simulink model "step_model"  (R2015b)
settings: Solver=VariableStepAuto  StartTime=0.0  StopTime=10.0  RelTol=1e-3
values from neighbouring files (symbols this model uses):
  A = [zeros(2) eye(2); -inv(M)*kappa -inv(M)*beta]    [Lab3_Solution.m]    (also in lab4.m = [0 0 1 0; 0 0 0 1; 0 (mp^2 * l^2 *g)/mu (-c*Jt)/mu (-Y*Jt*l*; lab4_pid_controller.m; lab4_state_feedback_no_estimator.m; lab4_state_feedback_with_estimator.m)
  B = [0; 0; inv(M)*S]    [Lab3_Solution.m]    (also in lab4.m = [0; 0; Jt/mu; (l*mp)/mu]; lab4_pid_controller.m; lab4_state_feedback_no_estimator.m; lab4_state_feedback_with_estimator.m)
  C = [1 0 0 0; 0 1 0 0]    [Lab3_Solution.m]    (also in PendulumTutorial.m = zpk(z,p,k); lab4.m; lab4_pid_controller.m; lab4_state_feedback_no_estimator.m = eye(4))
  D = [0; 0]    [Lab3_Solution.m]    (also in lab4.m; lab4_pid_controller.m; lab4_state_feedback_no_estimator.m = [0; 0; 0; 0]; lab4_state_feedback_with_estimator.m)
settings Model: Creator=lukasgemar  LastModifiedBy=lukasgemar

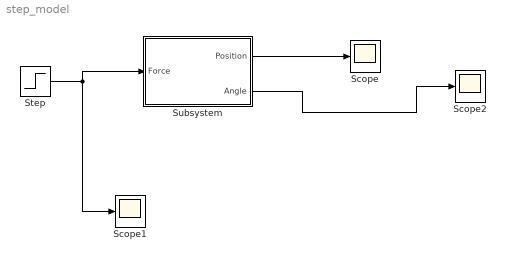
== system step_model ==
  Scope : Scope
  Scope1 : Scope
  Scope2 : Scope
  Step : Step  SampleTime=0
  Subsystem : Subsystem
  wires:
  Step/1 -> Subsystem/1(Force), Scope1/1
  Subsystem/1(Position) -> Scope/1
  Subsystem/2(Angle) -> Scope2/1

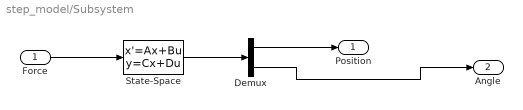
== system step_model/Subsystem ==
  Force : Inport
  Demux : Demux  Outputs=2
  State-Space : StateSpace  A=A  B=B  C=C  D=D  X0=0
  Position : Outport
  Angle : Outport  Port=2
  wires:
  State-Space/1 -> Demux/1
  Demux/2 -> Angle/1
  Force/1 -> State-Space/1
  Demux/1 -> Position/1
